simulink model "main"  (R2022a)
settings: Solver=FixedStepAuto  StartTime=0.0  StopTime=3  MaxStep=1e-6  RelTol=1e-3
values from neighbouring files (symbols this model uses):
  J = 0.0025    [params.m]
  Ka_c = 1/Kp_c    (= 1.32419455106)    [params.m]
  Ka_s = 1/Kp_s    (= 1.9123477716)    [params.m]
  Ki_c = Ra*wcc    (= 115.497512317)    [params.m]
  Ki_s = Kp_s*wcs/5    (= 9.291640523)    [params.m]
  Kp_c = La*wcc    (= 0.75517604207)    [params.m]
  Kp_s = J*wcs/Kt    (= 0.522917439416)    [params.m]
  Kt = Te_rated/Ia_rated    (= 0.424752712124)    [params.m]
  La = 1.7e-3    (= 0.0017)    [params.m]
  Ra = 0.26    [params.m]
  Te_rated = power_rated/wm_rated    (= 10.6188178031)    [params.m]
  TL = 1    [params.m]
  Tsw = 1/fsw    (= 0.001)    [params.m]
  Va_rated = 140    [params.m]
  Vdc = 200    [params.m]
libraries: spsDCMachineLib x1, spsDCVoltageSourceLib x1, spsUniversalBridgeLib x1, simulink x1, spspowerguiLib x1
settings Model: Creator=lzd  LastModifiedBy=lzd

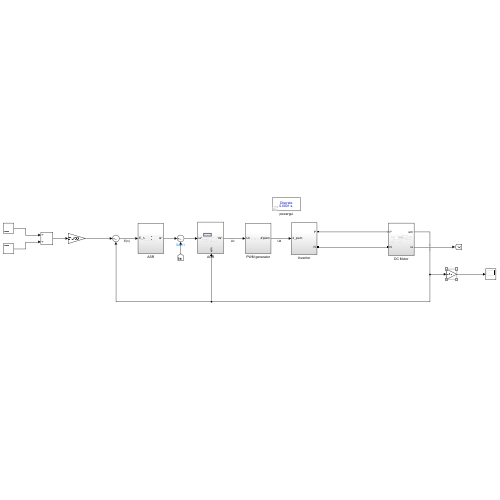
[thumbnail: Simulink's stored preview of the top-level diagram]
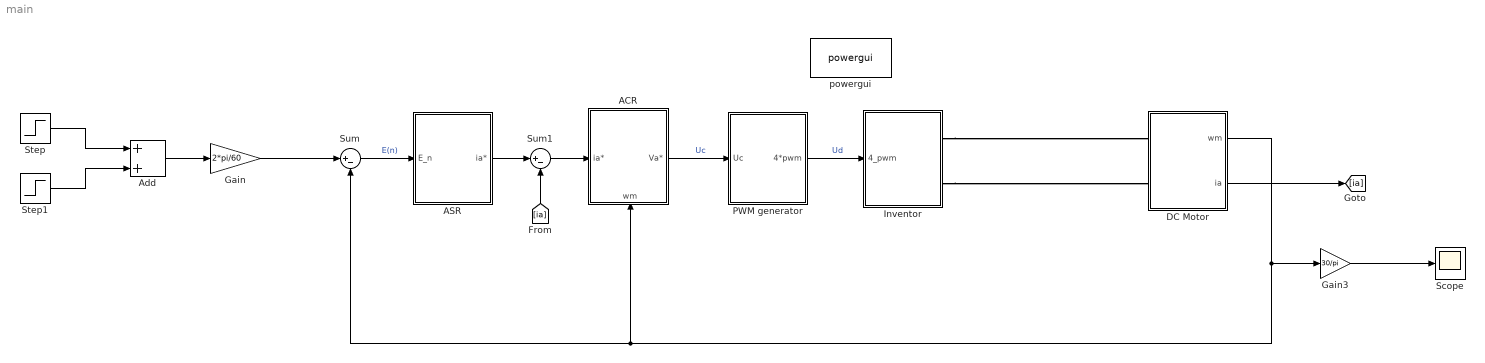
== system main ==
  ACR : Subsystem
      settings: PortSchema="{\"entries\":[{\"content\":{\"sides\":[{\"content\":{\"connectorIds\":[\"In1\"]},\"type\":\"ConnectorPlacement.EquallySpacedRectSide\",\"uuid\":\"3ee60535-b7ae-4158-b889-2a8b493230b2\"},{\"content\":{\"connectorIds\":[\"Out1\"],\"side\":\"RIGHT\"},\"type\":\"ConnectorPlacement.EquallySpacedRectSide\",\"uuid\":\"a9777d49-6c7a-4a4c-b166-bef4afe95680\"},{\"content\":{\"connectorIds\":[],\"side\":\"TOP\"},\"type\":\"ConnectorPlacement.EquallySpacedRectSide\",\"uuid\":\"f91be821-9ac9-4fe9-9bb0-fdf5df307c8b\"},{\"content\":{\"connectorIds\":[\"In2\"],\"side\":\"BOTTOM\"},\"type\":\"ConnectorPlacement.EquallySpacedRectSide\",\"uuid\":\"293d7cb4-f2eb-408b-bff2-b89237e8deb5\"}]},\"type\":\"ConnectorPlacement.EquallySpacedConnector\",\"uuid\":\"0b6413db-823d-4107-bd39-ec19c4fe0989\"}],\"packageUris\":[\"http://schema.mathworks.com/mf0/Connector/R2020b\"],\"version\":\"1.0\"}"
  ASR : Subsystem
  Add : Sum
  DC Motor : Subsystem
  Gain : Gain  Gain=2*pi/60
  Gain3 : Gain  Gain=30/pi
  Inventor : Subsystem
  PWM generator : Subsystem
  Scope : Scope
  Step : Step  Time=0  After=1000  SampleTime=0
  Step1 : Step  Time=2  After=-2000  SampleTime=0
  Sum : Sum  Inputs=|+-
  Sum1 : Sum  Inputs=|+-
  powergui : spspowerguiLib/powergui  Priority=1  SimulationMode=Discrete  SampleTime=Tsw/10  frequency=60  Iterations=50  frequencyindice=0  Pbase=100e6  ErrMax=1e-4  UnitsV=kV  UnitsW=MW  buscounter=0  FunctionMessages=off  echomessages=off  EnableUseOfTLC=off  CurrentSourceSwitches=off  DisableSnubberDevices=off  DisableRonSwitches=off  DisableVfSwitches=off  DisplayEquations=off  AutomaticDiscreteSolvers=off  SolverType=Tustin/Backward Euler (TBE)  Interpol=off  ExternalGateDelay=off  methode=off  Ts=100  x0status=blocks  SPID=on  SwTol=0  HookPort=off  NonlinearTolerance=1e-4  nMaxIteration=100  ContinueOnMaxIteration=off  RestoreLinks=warning  ResistiveCurrentMeasurement=off  Frange=[0:2:500]  Ylog=off  Xlog=on  ShowGrid=off  save=off  variable=ZData  structure=0  ZoomFFT=off  StartTime=0.0  cycles=1  DisplayStyle=1  fundamental=60  FreqAxis=off  MaxFrequency=1000  frequencyindicesteady=1  RmsSteady=1  display=off
  wires:
  Step/1 -> Add/1
  Step1/1 -> Add/2
  Sum/1 -> ASR/1(E_n)  "E(n)"
  DC Motor/1(wm) -> Sum/2, ACR/2(wm), Gain3/1
  ACR/1(Va*) -> PWM generator/1(Uc)  "Uc"
  PWM generator/1(4*pwm) -> Inventor/1(4_pwm)  "Ud"
  ASR/1(ia*) -> Sum1/1
  Sum1/1 -> ACR/1(ia*)
  [ia] -> Sum1/2
  DC Motor/2(ia) -> [ia]
  Add/1 -> Gain/1
  Gain/1 -> Sum/1
  Gain3/1 -> Scope/1
  connections:
  Inventor/RConn1 -- DC Motor/LConn1
  Inventor/RConn2 -- DC Motor/LConn2

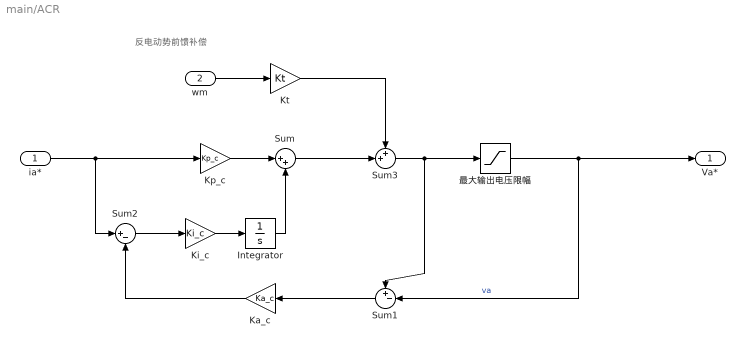
== system main/ACR ==
  note: 反电动势前馈补偿
  ia* : Inport
  wm : Inport  Port=2
  Integrator : Integrator
  Ka_c : Gain  Gain=Ka_c
  Ki_c : Gain  Gain=Ki_c
  Kp_c : Gain  Gain=Kp_c
  Kt : Gain  Gain=Kt
  Sum : Sum  Inputs=|++
  Sum1 : Sum  Inputs=+-|
  Sum2 : Sum  Inputs=|+-
  Sum3 : Sum  Inputs=++|
  最大输出电压限幅 : Saturate  UpperLimit=Va_rated  LowerLimit=-Va_rated
  Va* : Outport
  wires:
  Sum1/1 -> Ka_c/1
  Ki_c/1 -> Integrator/1
  Kp_c/1 -> Sum/1
  Integrator/1 -> Sum/2
  Sum2/1 -> Ki_c/1
  最大输出电压限幅/1 -> Va*/1, Sum1/2  "va"
  ia*/1 -> Sum2/1, Kp_c/1
  Ka_c/1 -> Sum2/2
  Kt/1 -> Sum3/1
  Sum/1 -> Sum3/2
  Sum3/1 -> Sum1/1, 最大输出电压限幅/1
  wm/1 -> Kt/1

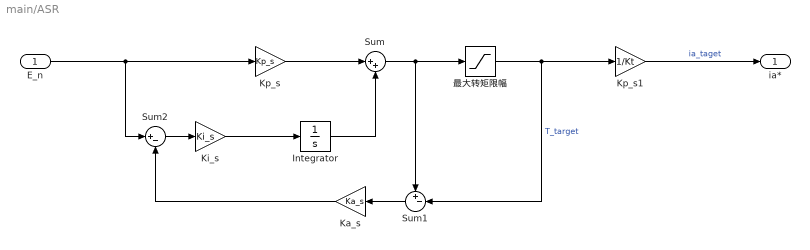
== system main/ASR ==
  E_n : Inport
  Integrator : Integrator
  Ka_s : Gain  Gain=Ka_s
  Ki_s : Gain  Gain=Ki_s
  Kp_s : Gain  Gain=Kp_s
  Kp_s1 : Gain  Gain=1/Kt
  Sum : Sum  Inputs=|++
  Sum1 : Sum  Inputs=+-|
  Sum2 : Sum  Inputs=|+-
  最大转矩限幅 : Saturate  UpperLimit=Te_rated  LowerLimit=-Te_rated
  ia* : Outport
  wires:
  E_n/1 -> Sum2/1, Kp_s/1
  Ki_s/1 -> Integrator/1
  Integrator/1 -> Sum/2
  Kp_s/1 -> Sum/1
  Sum/1 -> Sum1/1, 最大转矩限幅/1
  最大转矩限幅/1 -> Kp_s1/1, Sum1/2  "T_target"
  Sum1/1 -> Ka_s/1
  Ka_s/1 -> Sum2/2
  Sum2/1 -> Ki_s/1
  Kp_s1/1 -> ia*/1  "ia_taget"

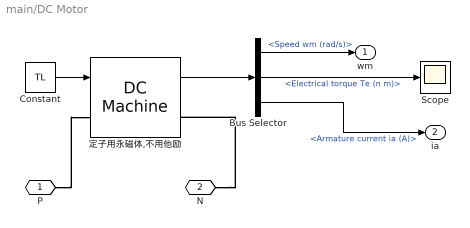
== system main/DC Motor ==
  Bus Selector : BusSelector  OutputSignals=Speed wm (rad/s),Electrical torque Te (n m),Armature current ia (A)
  Constant : Constant  Value=TL
  Scope : Scope
  定子用永磁体,不用他励 : spsDCMachineLib/DC Machine  PresetModel=No  MechanicalLoad=Torque TL  FieldType=Permanent magnet  ShowDetailedParameters=on  MeasurementBus=off  RLa=[Ra La]  RLf="[ 240  120]"  Laf=1.8  MachineConstant=Torque constant (N.m/A)  Ke=1.8  Kt=Kt  J=J  Bm=0  Tf=0  w0=0  Ifinit=1  TsPowergui=0  TsBlock=-1
  P : PMIOPort  Side=Left
  N : PMIOPort  Port=2  Side=Left
  wm : Outport
  ia : Outport  Port=2
  wires:
  定子用永磁体,不用他励/1 -> Bus Selector/1
  Bus Selector/1 -> wm/1  "<Speed wm (rad/s)>"
  Bus Selector/2 -> Scope/1  "<Electrical torque Te (n m)>"
  Bus Selector/3 -> ia/1  "<Armature current ia (A)>"
  Constant/1 -> 定子用永磁体,不用他励/1
  connections:
  P/RConn1 -- 定子用永磁体,不用他励/LConn1
  N/RConn1 -- 定子用永磁体,不用他励/RConn1

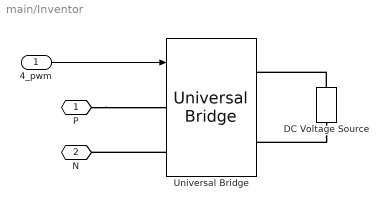
== system main/Inventor ==
  4_pwm : Inport
  DC Voltage Source : spsDCVoltageSourceLib/DC Voltage Source  Amplitude=Vdc  Measurements=None
  Universal Bridge : spsUniversalBridgeLib/Universal Bridge  Arms=2  SnubberResistance=1e5  SnubberCapacitance=inf  Device=IGBT / Diodes  Ron=1e-3  Lon=0  ForwardVoltages="[  0  0  ]"  ForwardVoltage=0  GTOparameters=[ 10e-6 , 20e-6 ]  IGBTparameters=[ 1e-6 , 2e-6 ]  Measurements=None  Measurements_2=None  converterType=Rectifier
  P : PMIOPort  Side=Right
  N : PMIOPort  Port=2  Side=Right
  wires:
  4_pwm/1 -> Universal Bridge/1
  connections:
  DC Voltage Source/RConn1 -- Universal Bridge/RConn1
  DC Voltage Source/LConn1 -- Universal Bridge/RConn2
  P/RConn1 -- Universal Bridge/LConn1
  Universal Bridge/LConn2 -- N/RConn1

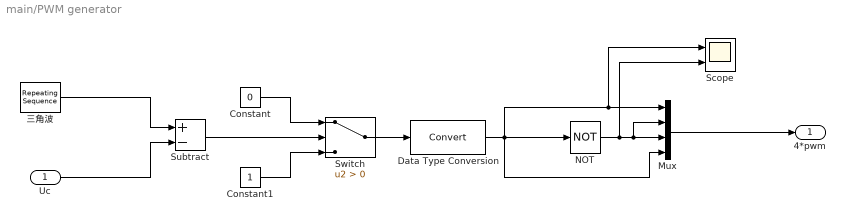
== system main/PWM generator ==
  Uc : Inport
  Constant : Constant  Value=0
  Constant1 : Constant
  Data Type Conversion : DataTypeConversion  SaturateOnIntegerOverflow=off  RndMeth=Floor
  Mux : Mux
  NOT : Logic  Operator=NOT  IconShape=distinctive  AllPortsSameDT=off  OutDataTypeStr=boolean
  Scope : Scope  NumInputPorts=2
  Subtract : Sum  Inputs=+-
  Switch : Switch  Criteria=u2 > Threshold  SaturateOnIntegerOverflow=off  InputSameDT=off
  三角波 : simulink/Sources/Repeating Sequence  rep_seq_t=[0 0.5*Tsw Tsw]  rep_seq_y=[-Vdc Vdc -Vdc]
  4*pwm : Outport
  wires:
  三角波/1 -> Subtract/1
  Uc/1 -> Subtract/2
  Subtract/1 -> Switch/2
  Constant/1 -> Switch/1
  Constant1/1 -> Switch/3
  Switch/1 -> Data Type Conversion/1
  Data Type Conversion/1 -> Mux/4, Scope/1, Mux/1, NOT/1
  NOT/1 -> Scope/2, Mux/3, Mux/2
  Mux/1 -> 4*pwm/1
